simulink model "Data_Type"  (Simulink 8.0)
settings: Solver=ode45  StartTime=0.0  StopTime=10.0  RelTol=1e-3
settings Model: Creator=Faradars  LastModifiedBy=Faradars

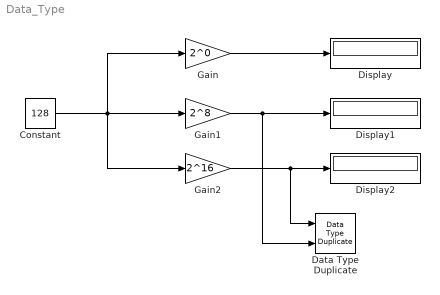
== system Data_Type ==
  Constant : Constant  Value=128
  Data Type Duplicate : DataTypeDuplicate
  Display : Display
  Display1 : Display
  Display2 : Display
  Gain : Gain  Gain=2^0
  Gain1 : Gain  Gain=2^8  OutDataTypeStr=double
  Gain2 : Gain  Gain=2^16  OutDataTypeStr=int8
  wires:
  Constant/1 -> Gain2/1, Gain/1, Gain1/1
  Gain/1 -> Display/1
  Gain1/1 -> Data Type Duplicate/2, Display1/1
  Gain2/1 -> Data Type Duplicate/1, Display2/1
